simulink model "BatteryPack4s"  (R2023b)
settings: Solver=VariableStepAuto  StartTime=0.0  StopTime=1369  RelTol=1e-3
undefined symbols (not defined in the file): Ion, Lithium
libraries: spsBatteryLib x12, spsControlledCurrentSourceLib x1, autolibshared x1, spsVoltageMeasurementLib x1, sps_lib x1
settings Model: Creator=marri  LastModifiedBy=marri
settings SolverCC: ZeroCrossAlgorithm=Adaptive
settings DebuggingCC: IgnoredZcDiagnostic=none

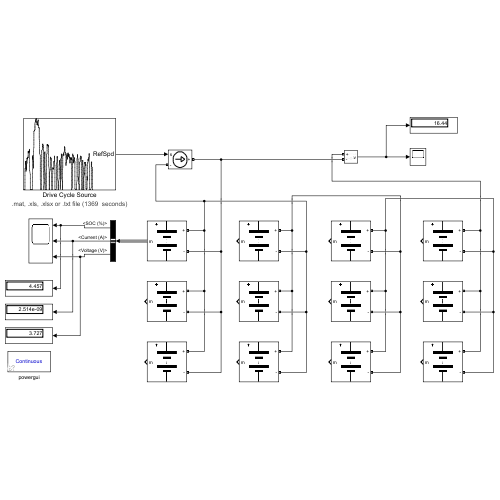
[thumbnail: Simulink's stored preview of the top-level diagram]
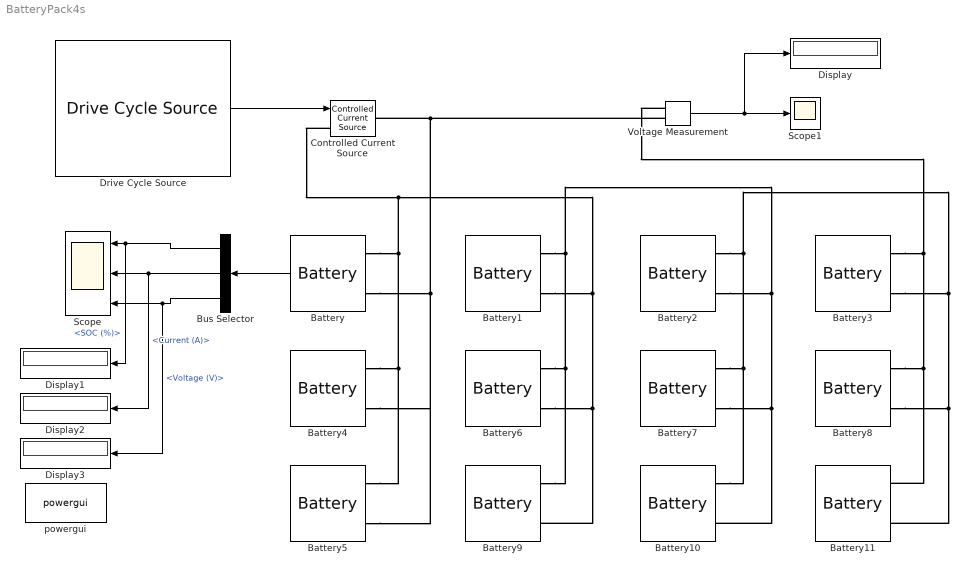
== system BatteryPack4s ==
  Battery{,1..11} (12 alike) : spsBatteryLib/Battery  BatType=Lithium-Ion  ShowTempParam=off  ThermalPreset=no  ShowAgeParam=off  NomV=3.7  NomQ=3  SOC=100  Batt_Tr=30  PresetModel=off  MaxQ=2.6  MinV=3.0  FullV=4.2  Dis_rate=0.52  R=0.07  Normal_OP=2.55  expZone="[4      0.4]"  current=[0.52 1.3 2.6]  Units=Time  Tci=20  NomT=20  T2=-30  MaxQ2=4.8  FullV2=7.1  Normal_OP2=5.655  expZone2="[6.58           1]"  Rca=0.6  ti=2000  Dp=0  Neq0=0  Tsim=1e6  Ta1=25  Qeol=5.4*0.9  Reol=0.013333*1.2  Char_age=[2.3478, 3]  Dis_age=[2.3478, 10]  N1=1500  N2=10500  N3=1000  N4=1400  Ta2=45  N5=950
  Bus Selector : BusSelector  OutputSignals=SOC (%),Current (A),Voltage (V)
  Controlled Current Source : spsControlledCurrentSourceLib/Controlled Current Source  Initialize=on  Source_Type=AC  Amplitude=0  Phase=0  Frequency=0  Measurements=None
  Display{,1..3} (4 alike) : Display
  Drive Cycle Source : autolibshared/Drive Cycle Source  cycleVar=.mat, .xls, .xlsx or .txt file  fileVar=E:\Matlab\Battery Modelling\DriveCycle.xlsx  tfinal="1369  seconds"  cycleRepeat=off  outAccPort=off  outGearPort=off  gearList=No gear data  t_wot1=5  xdot_woto=0  xdot_wot1=30  t_wot2=20  xdot_wot2=0  t_wotend=30  srcUnit=m/s  outUnit=m/s  srcAccUnit=m/s/s  outAccUnit=m/s^2  dt=0  aMode=1  faultOption=off  velBnd=2  velBndUnit=mph  inUnit=m/s  timeBnd=1  failOption=off  stopSim=off  maxFaultCnt=10  maxFaultTime=2  maxTotFaultTime=15  traceOption=off  dtTrace=1  traceWindow=10  lastDCname=Custom Data Set  lastOutUnit=mph  lastDT=0  lastTB=1  lastSB=2  forceCalcBound=off
  Scope : Scope  NumInputPorts=3
  Scope1 : Scope
  Voltage Measurement : spsVoltageMeasurementLib/Voltage Measurement  PhasorSimulation=off  OutputType=Complex  PSBequivalent=0
  powergui : sps_lib/powergui  Priority=1  SimulationMode=Continuous  SampleTime=50e-6  frequency=60  Iterations=50  frequencyindice=0  Pbase=100e6  ErrMax=1e-4  UnitsV=kV  UnitsW=MW  buscounter=0  FunctionMessages=off  echomessages=off  EnableUseOfTLC=off  CurrentSourceSwitches=off  DisableSnubberDevices=off  DisableRonSwitches=off  DisableVfSwitches=off  DisplayEquations=off  AutomaticDiscreteSolvers=off  SolverType=Tustin/Backward Euler (TBE)  Interpol=off  ExternalGateDelay=off  methode=off  Ts=100  x0status=blocks  SPID=on  SwTol=0  HookPort=off  NonlinearTolerance=1e-4  nMaxIteration=100  ContinueOnMaxIteration=off  RestoreLinks=warning  ResistiveCurrentMeasurement=off  Frange=[0:2:500]  Ylog=off  Xlog=on  ShowGrid=off  save=off  variable=ZData  structure=0  ZoomFFT=off  StartTime=0.0  cycles=1  DisplayStyle=1  fundamental=60  FreqAxis=off  MaxFrequency=1000  frequencyindicesteady=1  RmsSteady=1  display=off
  wires:
  Drive Cycle Source/1 -> Controlled Current Source/1
  Battery/1 -> Bus Selector/1
  Bus Selector/2 -> Scope/2, Display2/1  "<Current (A)>"
  Bus Selector/1 -> Display1/1, Scope/1  "<SOC (%)>"
  Bus Selector/3 -> Scope/3, Display3/1  "<Voltage (V)>"
  Voltage Measurement/1 -> Scope1/1, Display/1
  connections:
  Battery5/LConn1 -- Battery4/LConn1 -- Battery/LConn1 -- Controlled Current Source/LConn1 -- Battery1/LConn2 -- Battery6/LConn2 -- Battery9/LConn2
  Battery9/LConn1 -- Battery6/LConn1 -- Battery1/LConn1 -- Battery10/LConn2 -- Battery7/LConn2 -- Battery2/LConn2
  Battery10/LConn1 -- Battery3/LConn2 -- Battery11/LConn2 -- Battery8/LConn2 -- Battery2/LConn1 -- Battery7/LConn1
  Voltage Measurement/LConn2 -- Battery5/LConn2 -- Battery4/LConn2 -- Battery/LConn2 -- Controlled Current Source/RConn1
  Voltage Measurement/LConn1 -- Battery3/LConn1 -- Battery11/LConn1 -- Battery8/LConn1
